simulink model "MTQ_spin_test"  (R2016b)
settings: Solver=VariableStepAuto  StartTime=0.0  StopTime=10.0  RelTol=1e-3
libraries: dynamics_lib x1, environment_lib x1, bus_stubs_template x1
settings Model: Creator=taylorreynolds  LastModifiedBy=taylorreynolds

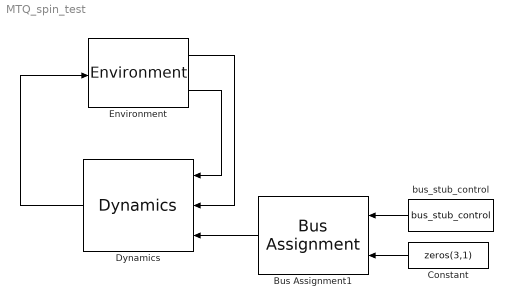
== system MTQ_spin_test ==
  Bus Assignment1 : BusAssignment  AssignedSignals=MT_dipole_Am2
  Constant : Constant  Value=zeros(3,1)
  Dynamics : dynamics_lib/Dynamics
  Environment : environment_lib/Environment
  bus_stub_control : bus_stubs_template/bus_stub_control
  wires:
  Dynamics/1 -> Environment/1
  Environment/2 -> Dynamics/1
  Environment/1 -> Dynamics/2
  Constant/1 -> Bus Assignment1/2
  Bus Assignment1/1 -> Dynamics/3
  bus_stub_control/1 -> Bus Assignment1/1
